simulink model "arlht_1920_1080"  (R2020a)
settings: Solver=FixedStepDiscrete  StartTime=0.0  StopTime=inf  RelTol=1e-3
InitFcn:
  | setup_parallel_hough_transform;
StopFcn:
  | %stop_parallel_hough_accumulator;
values from neighbouring files (symbols this model uses):
  bitsRho = ceil(log2(maxRho*2))    [setup_parallel_hough_transform.m]
  gamma = (179+1)/Ktheta    (= 45)    [setup_parallel_hough_transform.m]
  height = 1080    [setup_parallel_hough_transform.m]
  inarray = Y    [setup_parallel_hough_transform.m]
  Ktheta = 4    [setup_parallel_hough_transform.m]
  maxRho = ceil(sqrt((height/2)^2+(width/2)^2))    [setup_parallel_hough_transform.m]
  width = 1920    [setup_parallel_hough_transform.m]
undefined symbols (not defined in the file or in its folder): nTheta
libraries: simulink x27, hdlsllib x27, dspsrcs4 x1, dsphdlmathfun x1
(part 1 of 2)
settings Model: DataTypeOverride=Off  SimulationMode=rapid-accelerator  Creator=david  LastModifiedBy=david
settings OptimizationCC: BlockReduction=off  ConditionallyExecuteInputs=off  DefaultParameterBehavior=Inlined
settings DebuggingCC: AlgebraicLoopMsg=error  SingleTaskRateTransMsg=error
settings HardwareCC: ProdBitPerPointer=32  ProdBitPerSizeT=32  ProdBitPerPtrDiffT=32  ProdLargestAtomicFloat=None  ProdIntDivRoundTo=Undefined  ProdEndianess=Unspecified  ProdWordSize=32  ProdHWDeviceType=ASIC/FPGA->ASIC/FPGA  TargetBitPerPointer=64  TargetBitPerSizeT=64  TargetBitPerPtrDiffT=64  TargetLongLongMode=on  TargetIntDivRoundTo=Zero  TargetEndianess=LittleEndian  TargetWordSize=64  TargetHWDeviceType=Custom Processor->MATLAB Host Computer  ProdEqTarget=off

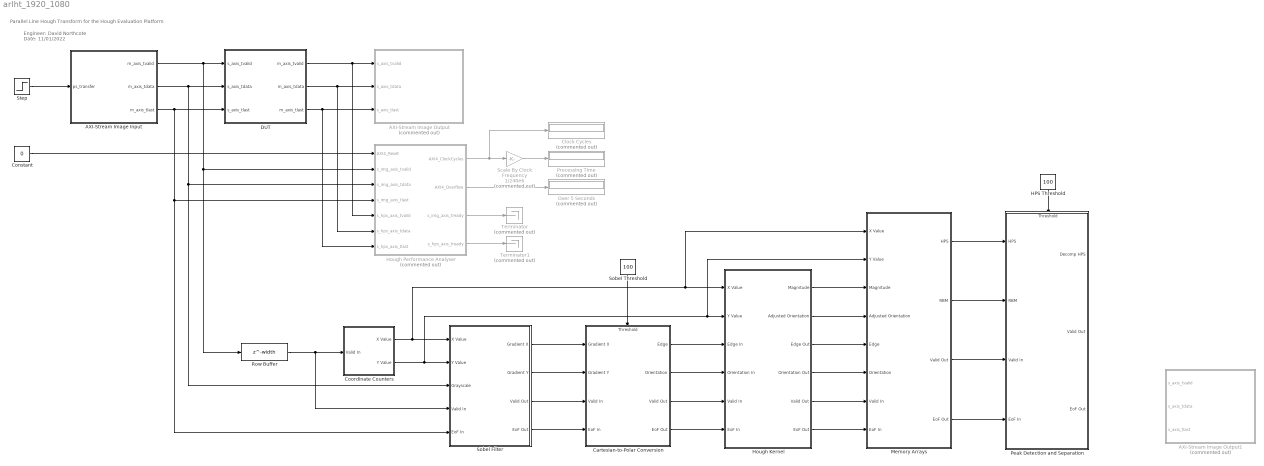
== system arlht_1920_1080 ==
  note: Engineer: David Northcote
      | Date: 11/01/2022
  note: Parallel Line Hough Transform for the Hough Evaluation Platform
  AXI-Stream Image Input : Subsystem  mask{image=inarray, clk=1/150e6}
      mask prompts: image "Input Image:"; clk "Clock Rate:"
      mask init:
      | [height, width] = size(image);
      mask DialogControl DescGroupVar Prompt: AXI-Stream Image Input
      mask DialogControl DescTextVar Prompt: This block simulates an AXI-Stream image input for interfacing to a hardware accelerator or IP Core.
      mask DialogControl ParameterGroupVar Prompt: Main
  AXI-Stream Image Output : Subsystem  Commented=on  mask{height=ceil(sqrt((height/2)^2+(width/2)^2))*2, width=numel([0:1:179]), clk=1/150e6, d=0}
      mask prompts: height "Image Height:"; width "Image Width:"; clk "Clock Rate:"; d "Frame Capture Number"
      mask DialogControl DescGroupVar Prompt: AXI-Stream Image Output
      mask DialogControl DescTextVar Prompt: Image output using the AXI-Stream interface. Simulates an AXI DMA write channel.
      mask DialogControl ParameterGroupVar Prompt: Main
  AXI-Stream Image Output1 : Subsystem  Commented=on  mask{height=height, width=width, clk=1/150e6, d=0}
      mask prompts: height "Image Height:"; width "Image Width:"; clk "Clock Rate:"; d "Frame Capture Number"
      mask DialogControl DescGroupVar Prompt: AXI-Stream Image Output
      mask DialogControl DescTextVar Prompt: Image output using the AXI-Stream interface. Simulates an AXI DMA write channel.
      mask DialogControl ParameterGroupVar Prompt: Main
  Cartesian-to-Polar Conversion : Subsystem
      settings: PortSchema="{\"entries\":[{\"content\":{\"sides\":[{\"content\":{\"connectorIds\":[\"In1\",\"In2\",\"In3\",\"In4\"]},\"type\":\"ConnectorPlacement.EquallySpacedRectSide\",\"uuid\":\"a3c8f507-c537-40f1-9a8a-bf401aec1e83\"},{\"content\":{\"connectorIds\":[\"Out1\",\"Out2\",\"Out3\",\"Out4\"],\"side\":\"RIGHT\"},\"type\":\"ConnectorPlacement.EquallySpacedRectSide\",\"uuid\":\"71853828-b65c-4dcd-97ef-062e77f4992b\"},{\"content\":{\"connectorIds\":[\"In5\"],\"side\":\"TOP\"},\"type\":\"ConnectorPlacement.EquallySpacedRectSide\",\"uuid\":\"70d50e18-3706-4f3a-b062-ad028f7ac4e8\"}]},\"type\":\"ConnectorPlacement.EquallySpacedConnector\",\"uuid\":\"ca8aacb5-c0af-4164-af92-5b8669b0f313\"}],\"packageUris\":[\"http://schema.mathworks.com/mf0/Connector/19700101\"],\"version\":\"1.0\"}"
  Clock Cycles : Display  Commented=on
  Constant : Constant  Value=0  OutDataTypeStr=boolean  SampleTime=1/150e6
  Coordinate Counters : Subsystem
  DUT : Subsystem  TreatAsAtomicUnit=on
  HPS Threshold : Constant  Value=100  OutDataTypeStr=uint8  SampleTime=-1
  Hough Kernel : Subsystem
  Hough Performance Analyser : Subsystem  Commented=on  TreatAsAtomicUnit=on
  Memory Arrays : Subsystem
  Over 5 Seconds : Display  Commented=on
  Peak Detection and Separation : Subsystem
      settings: PortSchema="{\"entries\":[{\"content\":{\"sides\":[{\"content\":{\"connectorIds\":[\"In1\",\"In2\",\"In3\",\"In4\"]},\"type\":\"ConnectorPlacement.EquallySpacedRectSide\",\"uuid\":\"a3c8f507-c537-40f1-9a8a-bf401aec1e83\"},{\"content\":{\"connectorIds\":[\"Out1\",\"Out2\",\"Out3\"],\"side\":\"RIGHT\"},\"type\":\"ConnectorPlacement.EquallySpacedRectSide\",\"uuid\":\"71853828-b65c-4dcd-97ef-062e77f4992b\"},{\"content\":{\"connectorIds\":[\"In5\"],\"side\":\"TOP\"},\"type\":\"ConnectorPlacement.EquallySpacedRectSide\",\"uuid\":\"70d50e18-3706-4f3a-b062-ad028f7ac4e8\"}]},\"type\":\"ConnectorPlacement.EquallySpacedConnector\",\"uuid\":\"ca8aacb5-c0af-4164-af92-5b8669b0f313\"}],\"packageUris\":[\"http://schema.mathworks.com/mf0/Connector/19700101\"],\"version\":\"1.0\"}"
  Processing Time : Display  Commented=on
  Row Buffer : Delay  DelayLength=width
  Scale By Clock Frequency : Gain  Commented=on  Gain=1/240e6  ParamDataTypeStr=double  OutDataTypeStr=double
  Sobel Filter : Subsystem
  Sobel Threshold : Constant  Value=100  OutDataTypeStr=uint8  SampleTime=-1
  Step : Step  Time=2/150e6  SampleTime=1/150e6
  Terminator : Terminator  Commented=on
  Terminator1 : Terminator  Commented=on
  wires:
  Hough Performance Analyser/1(AXI4_ClockCycles) -> Clock Cycles/1, Scale By Clock Frequency/1
  Scale By Clock Frequency/1 -> Processing Time/1
  DUT/3(m_axis_tlast) -> Hough Performance Analyser/7(s_hps_axis_tlast), AXI-Stream Image Output/3(s_axis_tlast)
  DUT/2(m_axis_tdata) -> Hough Performance Analyser/6(s_hps_axis_tdata), AXI-Stream Image Output/2(s_axis_tdata)
  DUT/1(m_axis_tvalid) -> Hough Performance Analyser/5(s_hps_axis_tvalid), AXI-Stream Image Output/1(s_axis_tvalid)
  AXI-Stream Image Input/3(m_axis_tlast) -> Sobel Filter/5(EoF In), Hough Performance Analyser/4(s_img_axis_tlast), DUT/3(s_axis_tlast)
  AXI-Stream Image Input/1(m_axis_tvalid) -> Row Buffer/1, Hough Performance Analyser/2(s_img_axis_tvalid), DUT/1(s_axis_tvalid)
  AXI-Stream Image Input/2(m_axis_tdata) -> Sobel Filter/3(Grayscale), Hough Performance Analyser/3(s_img_axis_tdata), DUT/2(s_axis_tdata)
  Hough Performance Analyser/2(AXI4_Overflow) -> Over 5 Seconds/1
  Constant/1 -> Hough Performance Analyser/1(AXI4_Reset)
  Step/1 -> AXI-Stream Image Input/1(ps_transfer)
  Hough Performance Analyser/4(s_hps_axis_tready) -> Terminator1/1
  Hough Performance Analyser/3(s_img_axis_tready) -> Terminator/1
  Coordinate Counters/2(Y Value) -> Memory Arrays/2(Y Value), Hough Kernel/2(Y Value), Sobel Filter/2(Y Value)
  Coordinate Counters/1(X Value) -> Hough Kernel/1(X Value), Memory Arrays/1(X Value), Sobel Filter/1(X Value)
  Row Buffer/1 -> Coordinate Counters/1(Valid In), Sobel Filter/4(Valid In)
  Sobel Filter/3(Valid Out) -> Cartesian-to-Polar Conversion/3(Valid In)
  Sobel Filter/4(EoF Out) -> Cartesian-to-Polar Conversion/4(EoF In)
  Sobel Filter/1(Gradient X) -> Cartesian-to-Polar Conversion/1(Gradient X)
  Sobel Filter/2(Gradient Y) -> Cartesian-to-Polar Conversion/2(Gradient Y)
  Cartesian-to-Polar Conversion/1(Edge) -> Hough Kernel/3(Edge In)
  Cartesian-to-Polar Conversion/2(Orientation) -> Hough Kernel/4(Orientation In)
  Cartesian-to-Polar Conversion/3(Valid Out) -> Hough Kernel/5(Valid In)
  Cartesian-to-Polar Conversion/4(EoF Out) -> Hough Kernel/6(EoF In)
  Hough Kernel/3(Edge Out) -> Memory Arrays/5(Edge)
  Hough Kernel/1(Magnitude) -> Memory Arrays/3(Magnitude)
  Hough Kernel/2(Adjusted Orientation) -> Memory Arrays/4(Adjusted Orientation)
  Hough Kernel/5(Valid Out) -> Memory Arrays/7(Valid In)
  Hough Kernel/6(EoF Out) -> Memory Arrays/8(EoF In)
  Sobel Threshold/1 -> Cartesian-to-Polar Conversion/5(Threshold)
  Memory Arrays/4(EoF Out) -> Peak Detection and Separation/4(EoF In)
  Memory Arrays/3(Valid Out) -> Peak Detection and Separation/3(Valid In)
  Memory Arrays/2(RBM) -> Peak Detection and Separation/2(RBM)
  Memory Arrays/1(HPS) -> Peak Detection and Separation/1(HPS)
  HPS Threshold/1 -> Peak Detection and Separation/5(Threshold)
  Hough Kernel/4(Orientation Out) -> Memory Arrays/6(Orientation)

== system arlht_1920_1080/AXI-Stream Image Input ==
  ps_transfer : Inport
  Compare To Constant : simulink/Logic and Bit Operations/Compare To Constant  relop===  const=height*width-1  OutDataTypeStr=boolean
  Constant : Constant  OutDataTypeStr=boolean  SampleTime=-1
  Data Type Conversion : DataTypeConversion  OutDataTypeStr=uint32
  HDL Counter : hdlsllib/Sources/HDL Counter  CountType=Free running  CountInit=0  CountStep=1  CountMax=width*height-1  CountFromType=Initial value  CountFrom=0  CountResetPort=on  CountLoadPort=off  CountEnbPort=on  CountDirPort=off  CountDataType=Unsigned  CountWordLen=32  CountFracLen=0  CountSampTime=1
  Multiport Switch : MultiPortSwitch  DataPortOrder=Zero-based contiguous  Inputs=2  zeroidx=on
  Rising Edge Detector : Subsystem
  Synchronous Image Source : Subsystem
  Unit Delay Resettable Synchronous : hdlsllib/Discrete/Unit Delay Resettable Synchronous  InitialCondition=0.0  SampleTime=-1
      settings: SourceProductBaseCode=SL
  m_axis_tvalid : Outport
  m_axis_tdata : Outport  Port=2
  m_axis_tlast : Outport  Port=3
  wires:
  Constant/1 -> Multiport Switch/3
  Rising Edge Detector/1(Output) -> Multiport Switch/1
  Unit Delay Resettable Synchronous/1 -> Multiport Switch/2
  ps_transfer/1 -> Rising Edge Detector/1(Input)
  Data Type Conversion/1 -> m_axis_tdata/1
  Compare To Constant/1 -> m_axis_tlast/1, HDL Counter/1, Unit Delay Resettable Synchronous/2
  Multiport Switch/1 -> m_axis_tvalid/1, Synchronous Image Source/Enable, HDL Counter/2, Unit Delay Resettable Synchronous/1
  Synchronous Image Source/1(Pixel) -> Data Type Conversion/1
  HDL Counter/1 -> Compare To Constant/1

== system arlht_1920_1080/AXI-Stream Image Output ==
  s_axis_tvalid : Inport
  s_axis_tdata : Inport  Port=2
  s_axis_tlast : Inport  Port=3
  Delay : Delay  DelayLength=4
  Delay1 : Delay  DelayLength=d  ShowEnablePort=on
      settings: InputPortMap=u0,e6
  Pixel to Workspace : Subsystem
  Stop Simulation2 : Stop
  wires:
  Delay/1 -> Stop Simulation2/1
  Delay1/1 -> Delay/1
  s_axis_tlast/1 -> Delay1/1, Delay1/2
  s_axis_tdata/1 -> Pixel to Workspace/1(Pixel In)
  s_axis_tvalid/1 -> Pixel to Workspace/Enable

== system arlht_1920_1080/AXI-Stream Image Output1 ==
  s_axis_tvalid : Inport
  s_axis_tdata : Inport  Port=2
  s_axis_tlast : Inport  Port=3
  Delay : Delay  DelayLength=4
  Delay1 : Delay  DelayLength=d  ShowEnablePort=on
      settings: InputPortMap=u0,e6
  Pixel to Workspace : Subsystem
  Stop Simulation2 : Stop
  wires:
  s_axis_tvalid/1 -> Pixel to Workspace/Enable
  s_axis_tdata/1 -> Pixel to Workspace/1(Pixel In)
  s_axis_tlast/1 -> Delay1/2, Delay1/1
  Delay1/1 -> Delay/1
  Delay/1 -> Stop Simulation2/1

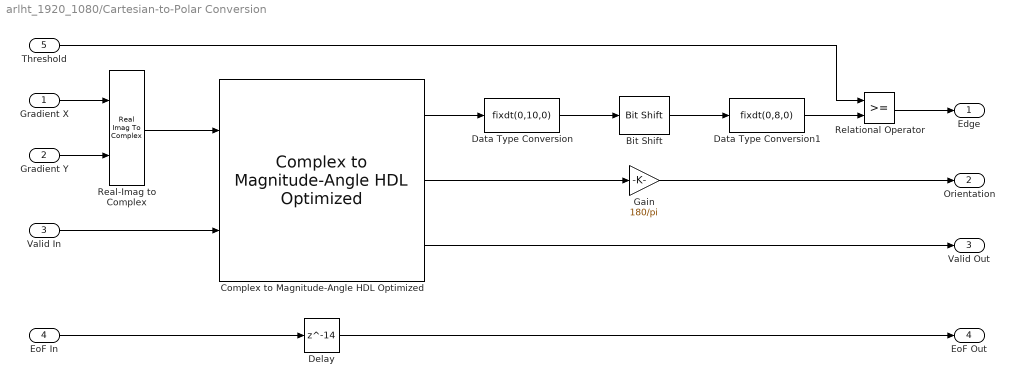
== system arlht_1920_1080/Cartesian-to-Polar Conversion ==
  Gradient X : Inport
  Gradient Y : Inport  Port=2
  Valid In : Inport  Port=3
  EoF In : Inport  Port=4
  Threshold : Inport  Port=5
  Bit Shift : hdlsllib/Logic and Bit Operations/Bit Shift  mode=Shift Right Logical  N=2
  Complex to Magnitude-Angle HDL Optimized : dsphdlmathfun/Complex to Magnitude-Angle HDL Optimized  NumIterationsSource=Property  NumIterations=9  OutputFormat=Magnitude and angle  AngleFormat=Radians  ScaleOutput=on  SimulateUsing=Code generation
      settings: SourceProductBaseCode=DS
  Data Type Conversion : DataTypeConversion  OutDataTypeStr=fixdt(0,10,0)  SaturateOnIntegerOverflow=on
  Data Type Conversion1 : DataTypeConversion  OutDataTypeStr=fixdt(0,8,0)  SaturateOnIntegerOverflow=on
  Delay : Delay  DelayLength=14
  Gain : Gain  Gain=180/pi  ParamDataTypeStr=fixdt(0,16,16-6)  OutDataTypeStr=uint8  RndMeth=Round
  Real-Imag to Complex : RealImagToComplex
  Relational Operator : RelationalOperator  OutDataTypeStr=boolean  RndMeth=Simplest
  Edge : Outport
  Orientation : Outport  Port=2
  Valid Out : Outport  Port=3
  EoF Out : Outport  Port=4
  wires:
  Real-Imag to Complex/1 -> Complex to Magnitude-Angle HDL Optimized/1
  Valid In/1 -> Complex to Magnitude-Angle HDL Optimized/2
  EoF In/1 -> Delay/1
  Complex to Magnitude-Angle HDL Optimized/3 -> Valid Out/1
  Delay/1 -> EoF Out/1
  Gradient X/1 -> Real-Imag to Complex/1
  Gradient Y/1 -> Real-Imag to Complex/2
  Complex to Magnitude-Angle HDL Optimized/1 -> Data Type Conversion/1
  Data Type Conversion/1 -> Bit Shift/1
  Bit Shift/1 -> Data Type Conversion1/1
  Complex to Magnitude-Angle HDL Optimized/2 -> Gain/1
  Gain/1 -> Orientation/1
  Data Type Conversion1/1 -> Relational Operator/2
  Relational Operator/1 -> Edge/1
  Threshold/1 -> Relational Operator/1

== system arlht_1920_1080/Coordinate Counters ==
  Valid In : Inport
  AND : Logic  IconShape=distinctive  AllPortsSameDT=off  OutDataTypeStr=boolean
  Compare To Constant : simulink/Logic and Bit Operations/Compare To Constant  relop===  const=width/2-1  OutDataTypeStr=boolean
  X Counter : hdlsllib/Sources/HDL Counter  CountType=Count limited  CountInit=-width/2  CountStep=1  CountMax=width/2-1  CountFromType=Initial value  CountFrom=-width/2  CountResetPort=off  CountLoadPort=off  CountEnbPort=on  CountDirPort=off  CountDataType=Signed  CountWordLen=ceil(log2(width/2)) + 1  CountFracLen=0  CountSampTime=1
  Y Counter : hdlsllib/Sources/HDL Counter  CountType=Count limited  CountInit=-height/2  CountStep=1  CountMax=height/2-1  CountFromType=Initial value  CountFrom=-height/2  CountResetPort=off  CountLoadPort=off  CountEnbPort=on  CountDirPort=off  CountDataType=Signed  CountWordLen=ceil(log2(height/2)) + 1  CountFracLen=0  CountSampTime=1
  X Value : Outport  VectorParamsAs1DForOutWhenUnconnected=off
  Y Value : Outport  Port=2  VectorParamsAs1DForOutWhenUnconnected=off
  wires:
  Valid In/1 -> AND/2, X Counter/1
  X Counter/1 -> X Value/1, Compare To Constant/1
  Y Counter/1 -> Y Value/1
  AND/1 -> Y Counter/1
  Compare To Constant/1 -> AND/1

== system arlht_1920_1080/DUT ==
  s_axis_tvalid : Inport
  s_axis_tdata : Inport  Port=2
  s_axis_tlast : Inport  Port=3
  LHT : Subsystem
  m_axis_tvalid : Outport  VectorParamsAs1DForOutWhenUnconnected=off
  m_axis_tdata : Outport  Port=2  VectorParamsAs1DForOutWhenUnconnected=off
  m_axis_tlast : Outport  Port=3  VectorParamsAs1DForOutWhenUnconnected=off
  wires:
  s_axis_tdata/1 -> LHT/1(s_tdata)
  s_axis_tvalid/1 -> LHT/2(s_tvalid)
  s_axis_tlast/1 -> LHT/3(s_tlast)
  LHT/3(m_axis_tlast) -> m_axis_tlast/1
  LHT/1(m_axis_tdata) -> m_axis_tdata/1
  LHT/2(m_axis_tvalid) -> m_axis_tvalid/1

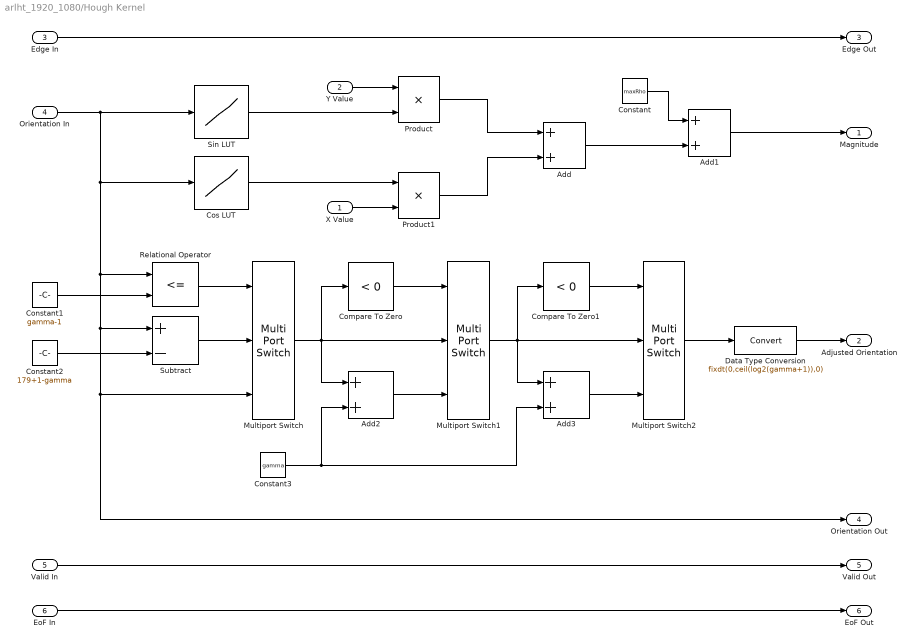
== system arlht_1920_1080/Hough Kernel ==
  X Value : Inport
  Y Value : Inport  Port=2
  Edge In : Inport  Port=3
  Orientation In : Inport  Port=4
  Valid In : Inport  Port=5
  EoF In : Inport  Port=6
  Add : Sum
  Add1 : Sum  OutDataTypeStr=fixdt(0,bitsRho,0)
  Add2 : Sum  OutDataTypeStr=Inherit: Same as first input
  Add3 : Sum  OutDataTypeStr=Inherit: Same as first input
  Compare To Zero : simulink/Logic and Bit Operations/Compare To Zero  relop=<  OutDataTypeStr=boolean
  Compare To Zero1 : simulink/Logic and Bit Operations/Compare To Zero  relop=<  OutDataTypeStr=boolean
  Constant : Constant  Value=maxRho  OutDataTypeStr=fixdt(0,ceil(log2(maxRho+1)),0)  SampleTime=-1
  Constant1 : Constant  Value=gamma-1  OutDataTypeStr=fixdt(0,ceil(log2(gamma)),0)  SampleTime=-1
  Constant2 : Constant  Value=179+1-gamma  OutDataTypeStr=fixdt(0,ceil(log2(179+1-gamma)),0)  SampleTime=-1
  Constant3 : Constant  Value=gamma  OutDataTypeStr=fixdt(0,ceil(log2(gamma+1)),0)  SampleTime=-1
  Cos LUT : Lookup_n-D  NumberOfTableDimensions=1  BreakpointsForDimension1=[0:1:179]  IndexSearchMethod=Evenly spaced points  Table=cos(deg2rad(0:1:179))  InterpMethod=Flat  DiagnosticForOutOfRangeInput=Error  InternalRulePriority=Speed  OutDataTypeStr=fixdt(1,16,14)  RndMeth=Simplest  InputSameDT=on
  Data Type Conversion : DataTypeConversion  OutDataTypeStr=fixdt(0,ceil(log2(gamma+1)),0)
  Multiport Switch : MultiPortSwitch  DataPortOrder=Zero-based contiguous  Inputs=2  zeroidx=on
  Multiport Switch1 : MultiPortSwitch  DataPortOrder=Zero-based contiguous  Inputs=2  zeroidx=on
  Multiport Switch2 : MultiPortSwitch  DataPortOrder=Zero-based contiguous  Inputs=2  zeroidx=on
  Product : Product  OutDataTypeStr=fixdt(1,ceil(log2(height)),0)  RndMeth=Round
  Product1 : Product  OutDataTypeStr=fixdt(1,ceil(log2(width)),0)  RndMeth=Round
  Relational Operator : RelationalOperator  Operator=<=  OutDataTypeStr=boolean  RndMeth=Simplest
  Sin LUT : Lookup_n-D  NumberOfTableDimensions=1  BreakpointsForDimension1=[0:1:179]  IndexSearchMethod=Evenly spaced points  Table=sin(deg2rad(0:1:179))  InterpMethod=Flat  DiagnosticForOutOfRangeInput=Error  InternalRulePriority=Speed  OutDataTypeStr=fixdt(1,16,14)  RndMeth=Simplest  InputSameDT=on
  Subtract : Sum  Inputs=+-
  Magnitude : Outport
  Adjusted Orientation : Outport  Port=2
  Edge Out : Outport  Port=3
  Orientation Out : Outport  Port=4
  Valid Out : Outport  Port=5
  EoF Out : Outport  Port=6
  wires:
  Valid In/1 -> Valid Out/1
  EoF In/1 -> EoF Out/1
  Edge In/1 -> Edge Out/1
  Sin LUT/1 -> Product/2
  Cos LUT/1 -> Product1/1
  Product/1 -> Add/1
  Product1/1 -> Add/2
  Y Value/1 -> Product/1
  X Value/1 -> Product1/2
  Orientation In/1 -> Sin LUT/1, Orientation Out/1, Multiport Switch/3, Subtract/1, Relational Operator/1, Cos LUT/1
  Add1/1 -> Magnitude/1
  Add/1 -> Add1/2
  Constant/1 -> Add1/1
  Relational Operator/1 -> Multiport Switch/1
  Constant1/1 -> Relational Operator/2
  Constant2/1 -> Subtract/2
  Constant3/1 -> Add3/2, Add2/2
  Multiport Switch/1 -> Add2/1, Compare To Zero/1, Multiport Switch1/2
  Add2/1 -> Multiport Switch1/3
  Compare To Zero/1 -> Multiport Switch1/1
  Subtract/1 -> Multiport Switch/2
  Compare To Zero1/1 -> Multiport Switch2/1
  Add3/1 -> Multiport Switch2/3
  Multiport Switch1/1 -> Add3/1, Compare To Zero1/1, Multiport Switch2/2
  Multiport Switch2/1 -> Data Type Conversion/1
  Data Type Conversion/1 -> Adjusted Orientation/1

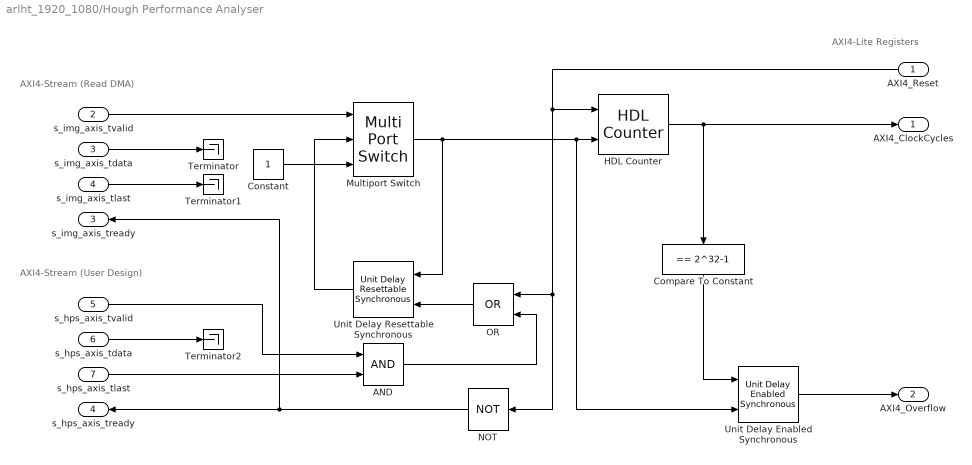
== system arlht_1920_1080/Hough Performance Analyser ==
  note: AXI4-Stream (Read DMA)
  note: AXI4-Stream (User Design)
  note: AXI4-Lite Registers
  AXI4_Reset : Inport
  s_img_axis_tvalid : Inport  Port=2
  s_img_axis_tdata : Inport  Port=3
  s_img_axis_tlast : Inport  Port=4
  s_hps_axis_tvalid : Inport  Port=5
  s_hps_axis_tdata : Inport  Port=6
  s_hps_axis_tlast : Inport  Port=7
  AND : Logic  IconShape=distinctive  AllPortsSameDT=off  OutDataTypeStr=boolean
  Compare To Constant : simulink/Logic and Bit Operations/Compare To Constant  relop===  const=2^32-1  OutDataTypeStr=boolean
  Constant : Constant  OutDataTypeStr=boolean  SampleTime=-1
  HDL Counter : hdlsllib/Sources/HDL Counter  CountType=Count limited  CountInit=0  CountStep=1  CountMax=2^32-1  CountFromType=Initial value  CountFrom=0  CountResetPort=on  CountLoadPort=off  CountEnbPort=on  CountDirPort=off  CountDataType=Unsigned  CountWordLen=32  CountFracLen=0  CountSampTime=1
  Multiport Switch : MultiPortSwitch  DataPortOrder=Zero-based contiguous  Inputs=2  zeroidx=on
  NOT : Logic  Operator=NOT  IconShape=distinctive  AllPortsSameDT=off  OutDataTypeStr=boolean
  OR : Logic  Operator=OR  IconShape=distinctive  AllPortsSameDT=off  OutDataTypeStr=boolean
  Terminator : Terminator
  Terminator1 : Terminator
  Terminator2 : Terminator
  Unit Delay Enabled Synchronous : hdlsllib/Discrete/Unit Delay Enabled Synchronous  InitialCondition=0.0  SampleTime=-1
      settings: SourceProductBaseCode=SL
  Unit Delay Resettable Synchronous : hdlsllib/Discrete/Unit Delay Resettable Synchronous  InitialCondition=0.0  SampleTime=-1
      settings: SourceProductBaseCode=SL
  AXI4_ClockCycles : Outport
  AXI4_Overflow : Outport  Port=2
  s_img_axis_tready : Outport  Port=3
  s_hps_axis_tready : Outport  Port=4
  wires:
  NOT/1 -> s_hps_axis_tready/1, s_img_axis_tready/1
  s_hps_axis_tvalid/1 -> AND/1
  s_hps_axis_tlast/1 -> AND/2
  AND/1 -> OR/2
  s_img_axis_tvalid/1 -> Multiport Switch/1
  OR/1 -> Unit Delay Resettable Synchronous/2
  s_img_axis_tlast/1 -> Terminator1/1
  AXI4_Reset/1 -> HDL Counter/1, OR/1, NOT/1
  s_img_axis_tdata/1 -> Terminator/1
  s_hps_axis_tdata/1 -> Terminator2/1
  HDL Counter/1 -> AXI4_ClockCycles/1, Compare To Constant/1
  Unit Delay Enabled Synchronous/1 -> AXI4_Overflow/1
  Compare To Constant/1 -> Unit Delay Enabled Synchronous/1
  Multiport Switch/1 -> HDL Counter/2, Unit Delay Enabled Synchronous/2, Unit Delay Resettable Synchronous/1
  Unit Delay Resettable Synchronous/1 -> Multiport Switch/2
  Constant/1 -> Multiport Switch/3

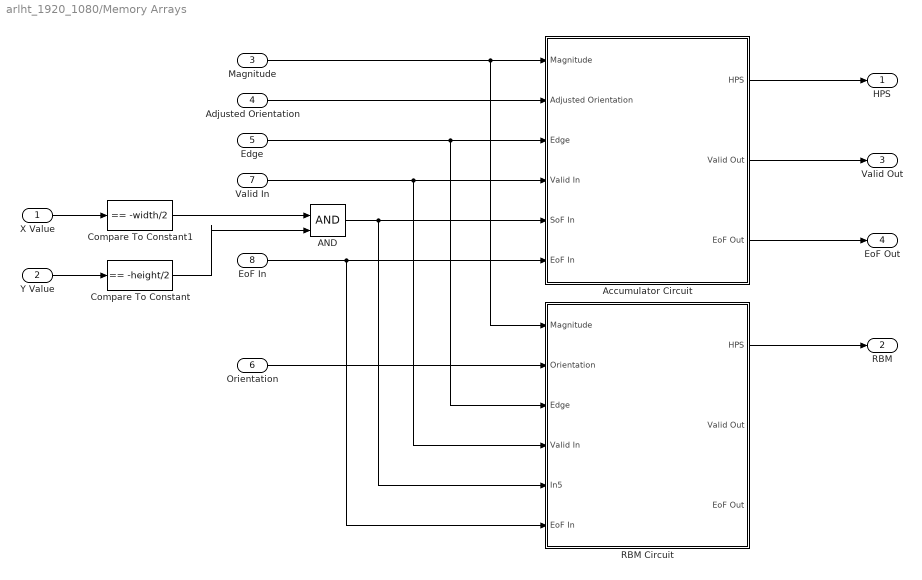
== system arlht_1920_1080/Memory Arrays ==
  X Value : Inport
  Y Value : Inport  Port=2
  Magnitude : Inport  Port=3
  Adjusted Orientation : Inport  Port=4
  Edge : Inport  Port=5
  Orientation : Inport  Port=6
  Valid In : Inport  Port=7
  EoF In : Inport  Port=8
  AND : Logic  IconShape=distinctive  AllPortsSameDT=off  OutDataTypeStr=boolean
  Accumulator Circuit : Subsystem
  Compare To Constant : simulink/Logic and Bit Operations/Compare To Constant  relop===  const=-height/2  OutDataTypeStr=boolean
  Compare To Constant1 : simulink/Logic and Bit Operations/Compare To Constant  relop===  const=-width/2  OutDataTypeStr=boolean
  RBM Circuit : Subsystem
  HPS : Outport
  RBM : Outport  Port=2
  Valid Out : Outport  Port=3
  EoF Out : Outport  Port=4
  wires:
  Magnitude/1 -> RBM Circuit/1(Magnitude), Accumulator Circuit/1(Magnitude)
  Adjusted Orientation/1 -> Accumulator Circuit/2(Adjusted Orientation)
  Edge/1 -> RBM Circuit/3(Edge), Accumulator Circuit/3(Edge)
  Valid In/1 -> RBM Circuit/4(Valid In), Accumulator Circuit/4(Valid In)
  EoF In/1 -> RBM Circuit/6(EoF In), Accumulator Circuit/6(EoF In)
  Accumulator Circuit/1(HPS) -> HPS/1
  RBM Circuit/1(HPS) -> RBM/1
  Accumulator Circuit/2(Valid Out) -> Valid Out/1
  Accumulator Circuit/3(EoF Out) -> EoF Out/1
  Orientation/1 -> RBM Circuit/2(Orientation)
  Compare To Constant/1 -> AND/2
  Compare To Constant1/1 -> AND/1
  X Value/1 -> Compare To Constant1/1
  Y Value/1 -> Compare To Constant/1
  AND/1 -> RBM Circuit/5(In5), Accumulator Circuit/5(SoF In)

== system arlht_1920_1080/Peak Detection and Separation ==
  HPS : Inport
  RBM : Inport  Port=2
  Valid In : Inport  Port=3
  EoF In : Inport  Port=4
  Threshold : Inport  Port=5
  Decomp HPS : Outport
  Valid Out : Outport  Port=2
  EoF Out : Outport  Port=3
  wires:
  ? -> Decomp HPS/1

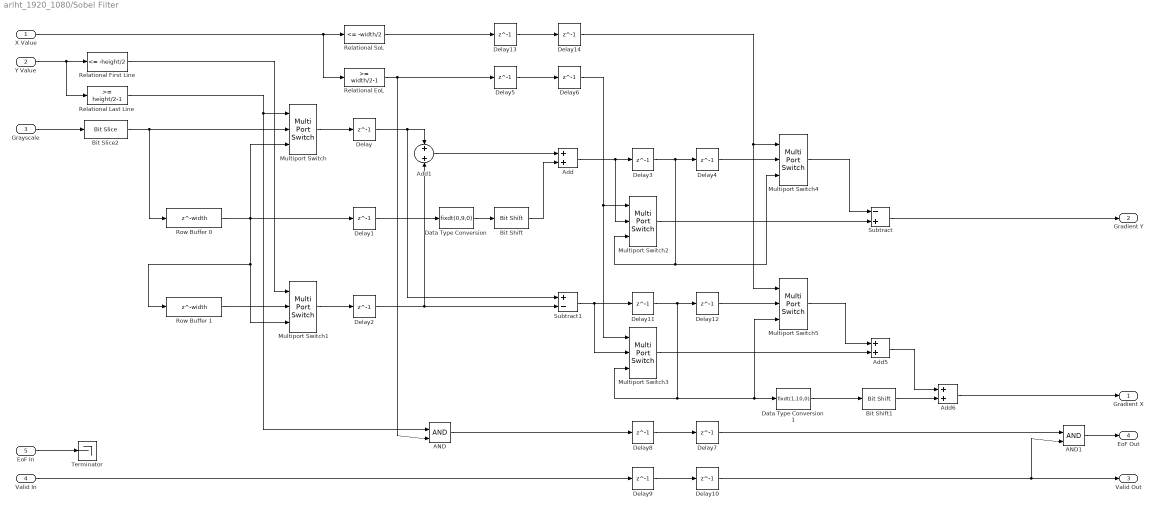
== system arlht_1920_1080/Sobel Filter ==
  X Value : Inport
  Y Value : Inport  Port=2
  Grayscale : Inport  Port=3
  Valid In : Inport  Port=4
  EoF In : Inport  Port=5
  AND : Logic  IconShape=distinctive  AllPortsSameDT=off  OutDataTypeStr=boolean
  AND1 : Logic  IconShape=distinctive  AllPortsSameDT=off  OutDataTypeStr=boolean
  Add{,1,5..6} (4 alike) : Sum
  Bit Shift : hdlsllib/Logic and Bit Operations/Bit Shift  mode=Shift Left Logical  N=1
  Bit Shift1 : hdlsllib/Logic and Bit Operations/Bit Shift  mode=Shift Left Logical  N=1
  Bit Slice2 : hdlsllib/Logic and Bit Operations/Bit Slice  lidx=7  ridx=0
      settings: SourceProductBaseCode=SL
  Data Type Conversion : DataTypeConversion  OutDataTypeStr=fixdt(0,9,0)
  Data Type Conversion1 : DataTypeConversion  OutDataTypeStr=fixdt(1,10,0)
  Delay{,1..14} (15 alike) : Delay  DelayLength=1
  Multiport Switch{,1..5} (6 alike) : MultiPortSwitch  DataPortOrder=Zero-based contiguous  Inputs=2  zeroidx=on
  Relational EoL : simulink/Logic and Bit Operations/Compare To Constant  relop=>=  const=width/2-1  OutDataTypeStr=boolean
  Relational First Line : simulink/Logic and Bit Operations/Compare To Constant  relop=<=  const=-height/2  OutDataTypeStr=boolean
  Relational Last Line : simulink/Logic and Bit Operations/Compare To Constant  relop=>=  const=height/2-1  OutDataTypeStr=boolean
  Relational SoL : simulink/Logic and Bit Operations/Compare To Constant  relop=<=  const=-width/2  OutDataTypeStr=boolean
  Row Buffer 0 : Delay  DelayLength=width
  Row Buffer 1 : Delay  DelayLength=width
  Subtract : Sum  Inputs=-+
  Subtract1 : Sum  Inputs=+-
  Terminator : Terminator
  Gradient X : Outport
  Gradient Y : Outport  Port=2
  Valid Out : Outport  Port=3
  EoF Out : Outport  Port=4
  wires:
  Grayscale/1 -> Bit Slice2/1
  Bit Slice2/1 -> Multiport Switch/2, Row Buffer 0/1
  EoF In/1 -> Terminator/1
  Add6/1 -> Gradient X/1
  Delay8/1 -> Delay7/1
  AND/1 -> Delay8/1
  Valid In/1 -> Delay9/1
  Delay9/1 -> Delay10/1
  Delay10/1 -> AND1/2, Valid Out/1
  Delay3/1 -> Multiport Switch2/3, Multiport Switch4/3, Delay4/1
  Data Type Conversion/1 -> Bit Shift/1
  Delay/1 -> Add1/1, Subtract1/1
  Add1/1 -> Add/1
  Delay1/1 -> Data Type Conversion/1
  Subtract/1 -> Gradient Y/1
  Delay2/1 -> Subtract1/2, Add1/2
  Delay11/1 -> Delay12/1, Multiport Switch3/3, Data Type Conversion1/1, Multiport Switch5/3
  Add5/1 -> Add6/1
  Bit Shift1/1 -> Add6/2
  Y Value/1 -> Relational Last Line/1, Relational First Line/1
  X Value/1 -> Relational EoL/1, Relational SoL/1
  Multiport Switch/1 -> Delay/1
  Relational Last Line/1 -> AND/1, Multiport Switch/1
  Multiport Switch1/1 -> Delay2/1
  Relational First Line/1 -> Multiport Switch1/1
  Row Buffer 0/1 -> Row Buffer 1/1, Multiport Switch1/3, Delay1/1, Multiport Switch/3
  Row Buffer 1/1 -> Multiport Switch1/2
  Multiport Switch2/1 -> Subtract/2
  Add/1 -> Delay3/1, Multiport Switch2/2
  Subtract1/1 -> Delay11/1, Multiport Switch3/2
  Multiport Switch3/1 -> Add5/2
  Relational EoL/1 -> AND/2, Delay5/1
  Delay5/1 -> Delay6/1
  Delay6/1 -> Multiport Switch2/1, Multiport Switch3/1
  Delay4/1 -> Multiport Switch4/2
  Multiport Switch4/1 -> Subtract/1
  Delay12/1 -> Multiport Switch5/2
  Multiport Switch5/1 -> Add5/1
  Relational SoL/1 -> Delay13/1
  Delay13/1 -> Delay14/1
  Delay14/1 -> Multiport Switch5/1, Multiport Switch4/1
  Delay7/1 -> AND1/1
  AND1/1 -> EoF Out/1
  Bit Shift/1 -> Add/2
  Data Type Conversion1/1 -> Bit Shift1/1

== system arlht_1920_1080/AXI-Stream Image Input/Rising Edge Detector ==
  Input : Inport
  AND : Logic  IconShape=distinctive  AllPortsSameDT=off  OutDataTypeStr=boolean
  Delay : Delay  DelayLength=1
  NOT : Logic  Operator=NOT  IconShape=distinctive  AllPortsSameDT=off  OutDataTypeStr=boolean
  Output : Outport  VectorParamsAs1DForOutWhenUnconnected=off
  wires:
  AND/1 -> Output/1
  Delay/1 -> AND/1
  Input/1 -> NOT/1, AND/2
  NOT/1 -> Delay/1

== system arlht_1920_1080/AXI-Stream Image Input/Synchronous Image Source ==
  Enable : EnablePort
  Signal From Workspace : dspsrcs4/Signal From Workspace  X=reshape(image', [height*width, 1])  Ts=clk  nsamps=1  OutputAfterFinalValue=Cyclic repetition  ignoreOrWarnInputAndFrameLengths=off  OutputFrames=off
  Pixel : Outport
  wires:
  Signal From Workspace/1 -> Pixel/1

== system arlht_1920_1080/AXI-Stream Image Output/Pixel to Workspace ==
  Pixel In : Inport
  Enable : EnablePort
  To Workspace : ToWorkspace  VariableName=simout  SampleTime=-1
      settings: MaxDataPoints=height*width  Save2DSignal=2-D array (concatenate along first dimension)
  wires:
  Pixel In/1 -> To Workspace/1

== system arlht_1920_1080/AXI-Stream Image Output1/Pixel to Workspace ==
  Pixel In : Inport
  Enable : EnablePort
  To Workspace : ToWorkspace  VariableName=simout  SampleTime=-1
      settings: MaxDataPoints=height*width  Save2DSignal=2-D array (concatenate along first dimension)
  wires:
  Pixel In/1 -> To Workspace/1

== system arlht_1920_1080/DUT/LHT ==
  s_tdata : Inport
  s_tvalid : Inport  Port=2
  s_tlast : Inport  Port=3
  Data Type Conversion : DataTypeConversion  Commented=on  OutDataTypeStr=uint32
  Parallel LHT Accumulator : Subsystem  Commented=on  mask{height=height, width=width, theta=[0:1:179]}
      mask prompts: height "Image Height:"; width "Image Width:"; theta "Orientations:"
      mask init:
      | maxRho = ceil(sqrt((height/2)^2+(width/2)^2));
      | nRho = maxRho*2;
      | [~, nTheta] = size(theta);
      mask DialogControl ParameterGroupVar Prompt: Main
  Parallel LHT Kernel : Subsystem  Commented=on
  m_axis_tdata : Outport  VectorParamsAs1DForOutWhenUnconnected=off
  m_axis_tvalid : Outport  Port=2  VectorParamsAs1DForOutWhenUnconnected=off
  m_axis_tlast : Outport  Port=3  VectorParamsAs1DForOutWhenUnconnected=off
  wires:
  s_tdata/1 -> Parallel LHT Kernel/1(s_tdata)
  s_tvalid/1 -> Parallel LHT Kernel/2(s_tvalid)
  s_tlast/1 -> Parallel LHT Kernel/3(s_tlast)
  Parallel LHT Kernel/1(m_axis_tvalid) -> Parallel LHT Accumulator/1(s_axis_tvalid)
  Parallel LHT Kernel/2(m_axis_tdata) -> Parallel LHT Accumulator/2(s_axis_tdata)
  Parallel LHT Kernel/4(m_axis_tlast) -> Parallel LHT Accumulator/4(s_axis_tlast)
  Parallel LHT Kernel/3(m_axis_tuser) -> Parallel LHT Accumulator/3(s_axis_tuser)
  Parallel LHT Kernel/5(hough_param) -> Parallel LHT Accumulator/5(hough_param)
  Parallel LHT Accumulator/2(m_axis_tdata) -> Data Type Conversion/1
  Parallel LHT Accumulator/1(m_axis_tvalid) -> m_axis_tvalid/1
  Parallel LHT Accumulator/3(m_axis_tlast) -> m_axis_tlast/1
  Data Type Conversion/1 -> m_axis_tdata/1

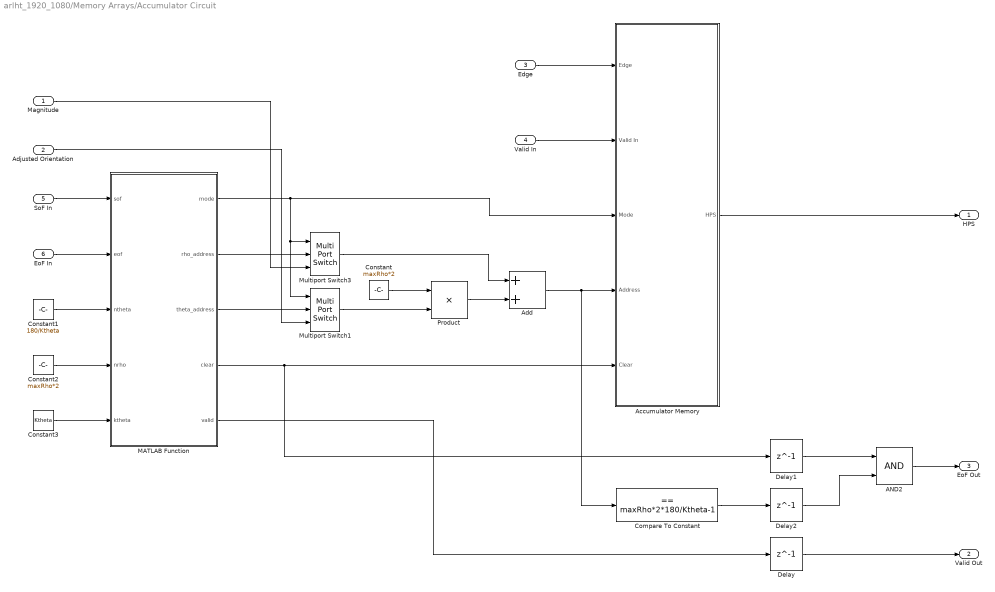
== system arlht_1920_1080/Memory Arrays/Accumulator Circuit ==
  Magnitude : Inport
  Adjusted Orientation : Inport  Port=2
  Edge : Inport  Port=3
  Valid In : Inport  Port=4
  SoF In : Inport  Port=5
  EoF In : Inport  Port=6
  AND2 : Logic  IconShape=distinctive  AllPortsSameDT=off  OutDataTypeStr=boolean
  Accumulator Memory : Subsystem
  Add : Sum  OutDataTypeStr=fixdt(0,ceil(log2(maxRho*2*45)),0)
  Compare To Constant : simulink/Logic and Bit Operations/Compare To Constant  relop===  const=maxRho*2*180/Ktheta-1  OutDataTypeStr=boolean
  Constant : Constant  Value=maxRho*2  OutDataTypeStr=fixdt(0,ceil(log2(maxRho*2+1)),0)  SampleTime=-1
  Constant1 : Constant  Value=180/Ktheta  OutDataTypeStr=uint8  SampleTime=-1
  Constant2 : Constant  Value=maxRho*2  OutDataTypeStr=uint16  SampleTime=-1
  Constant3 : Constant  Value=Ktheta  OutDataTypeStr=uint8  SampleTime=-1
  Delay : Delay  DelayLength=1  InitialCondition=0  UseCircularBuffer=on
  Delay1 : Delay  DelayLength=1  InitialCondition=0  UseCircularBuffer=on
  Delay2 : Delay  DelayLength=1  InitialCondition=0  UseCircularBuffer=on
  MATLAB Function : MATLAB Function  TreatAsAtomicUnit=on
  Multiport Switch1 : MultiPortSwitch  DataPortOrder=Zero-based contiguous  Inputs=2  zeroidx=on
  Multiport Switch3 : MultiPortSwitch  DataPortOrder=Zero-based contiguous  Inputs=2  zeroidx=on
  Product : Product  OutDataTypeStr=fixdt(0,ceil(log2(maxRho*2*44)),0)
  HPS : Outport
  Valid Out : Outport  Port=2
  EoF Out : Outport  Port=3
  wires:
  EoF In/1 -> MATLAB Function/2(eof)
  SoF In/1 -> MATLAB Function/1(sof)
  MATLAB Function/4(clear) -> Delay1/1, Accumulator Memory/5(Clear)
  MATLAB Function/5(valid) -> Delay/1
  Delay/1 -> Valid Out/1
  AND2/1 -> EoF Out/1
  Delay1/1 -> AND2/1
  Delay2/1 -> AND2/2
  Constant1/1 -> MATLAB Function/3(ntheta)
  Constant2/1 -> MATLAB Function/4(nrho)
  Constant3/1 -> MATLAB Function/5(ktheta)
  Compare To Constant/1 -> Delay2/1
  Magnitude/1 -> Multiport Switch3/3
  Adjusted Orientation/1 -> Multiport Switch1/3
  Edge/1 -> Accumulator Memory/1(Edge)
  Valid In/1 -> Accumulator Memory/2(Valid In)
  Accumulator Memory/1(HPS) -> HPS/1
  Add/1 -> Compare To Constant/1, Accumulator Memory/4(Address)
  Multiport Switch1/1 -> Product/2
  Multiport Switch3/1 -> Add/1
  Product/1 -> Add/2
  Constant/1 -> Product/1
  MATLAB Function/1(mode) -> Multiport Switch1/1, Multiport Switch3/1, Accumulator Memory/3(Mode)
  MATLAB Function/2(rho_address) -> Multiport Switch3/2
  MATLAB Function/3(theta_address) -> Multiport Switch1/2

== system arlht_1920_1080/Memory Arrays/RBM Circuit ==
  Magnitude : Inport
  Orientation : Inport  Port=2
  Edge : Inport  Port=3
  Valid In : Inport  Port=4
  In5 : Inport  Port=5
  EoF In : Inport  Port=6
  RBM Controller : Subsystem
  RBM Memory : Subsystem
  HPS : Outport
  Valid Out : Outport  Port=2
  EoF Out : Outport  Port=3
  wires:
  RBM Memory/1(hps) -> HPS/1
  RBM Controller/3(Out2) -> RBM Memory/3(enable)
  RBM Controller/2(y) -> RBM Memory/2(address)
  RBM Controller/1(Out1) -> RBM Memory/1(mode)
  RBM Controller/5(EoF Out) -> EoF Out/1
  RBM Controller/4(Valid Out) -> Valid Out/1
  EoF In/1 -> RBM Controller/5(EoF In)
  Valid In/1 -> RBM Controller/4(Valid In)
  Edge/1 -> RBM Controller/3(Edge)
  Orientation/1 -> RBM Controller/2(Adjusted Orientation)
  Magnitude/1 -> RBM Controller/1(Magnitude)

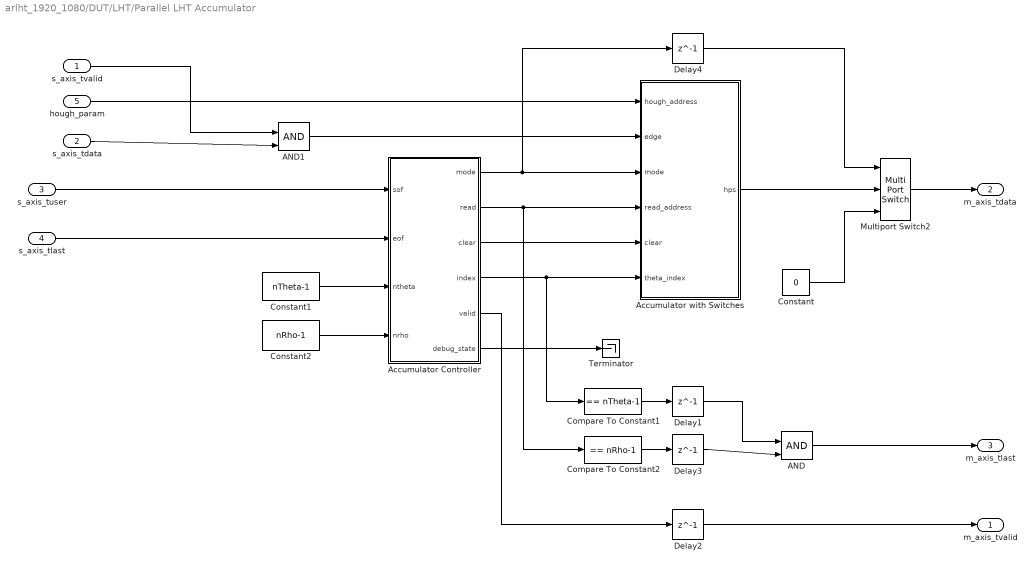
== system arlht_1920_1080/DUT/LHT/Parallel LHT Accumulator ==
  s_axis_tvalid : Inport
  s_axis_tdata : Inport  Port=2
  s_axis_tuser : Inport  Port=3
  s_axis_tlast : Inport  Port=4
  hough_param : Inport  Port=5
  AND : Logic  IconShape=distinctive  AllPortsSameDT=off  OutDataTypeStr=boolean
  AND1 : Logic  IconShape=distinctive  AllPortsSameDT=off  OutDataTypeStr=boolean
  Accumulator Controller : MATLAB Function  TreatAsAtomicUnit=on
  Accumulator with Switches : Subsystem
  Compare To Constant1 : simulink/Logic and Bit Operations/Compare To Constant  relop===  const=nTheta-1  OutDataTypeStr=boolean
  Compare To Constant2 : simulink/Logic and Bit Operations/Compare To Constant  relop===  const=nRho-1  OutDataTypeStr=boolean
  Constant : Constant  Value=0  OutDataTypeStr=fixdt(0, ceil(log2(2*maxRho)), 0)  SampleTime=-1
  Constant1 : Constant  Value=nTheta-1  OutDataTypeStr=uint16  SampleTime=-1
  Constant2 : Constant  Value=nRho-1  OutDataTypeStr=uint16  SampleTime=-1
  Delay{1..4} (4 alike) : Delay  DelayLength=1
  Multiport Switch2 : MultiPortSwitch  DataPortOrder=Zero-based contiguous  Inputs=2  zeroidx=on
  Terminator : Terminator
  m_axis_tvalid : Outport
  m_axis_tdata : Outport  Port=2
  m_axis_tlast : Outport  Port=3
  wires:
  s_axis_tlast/1 -> Accumulator Controller/2(eof)
  Accumulator Controller/6(debug_state) -> Terminator/1
  Delay4/1 -> Multiport Switch2/1
  Delay2/1 -> m_axis_tvalid/1
  Accumulator Controller/5(valid) -> Delay2/1
  Constant/1 -> Multiport Switch2/3
  Accumulator with Switches/1(hps) -> Multiport Switch2/2
  Multiport Switch2/1 -> m_axis_tdata/1
  s_axis_tvalid/1 -> AND1/1
  AND1/1 -> Accumulator with Switches/2(edge)
  s_axis_tdata/1 -> AND1/2
  hough_param/1 -> Accumulator with Switches/1(hough_address)
  s_axis_tuser/1 -> Accumulator Controller/1(sof)
  Constant2/1 -> Accumulator Controller/4(nrho)
  Compare To Constant2/1 -> Delay3/1
  Accumulator Controller/4(index) -> Compare To Constant1/1, Accumulator with Switches/6(theta_index)
  Constant1/1 -> Accumulator Controller/3(ntheta)
  Accumulator Controller/2(read) -> Accumulator with Switches/4(read_address), Compare To Constant2/1
  Accumulator Controller/1(mode) -> Accumulator with Switches/3(mode), Delay4/1
  Accumulator Controller/3(clear) -> Accumulator with Switches/5(clear)
  Compare To Constant1/1 -> Delay1/1
  Delay3/1 -> AND/2
  Delay1/1 -> AND/1
  AND/1 -> m_axis_tlast/1

== system arlht_1920_1080/DUT/LHT/Parallel LHT Kernel ==
  s_tdata : Inport
  s_tvalid : Inport  Port=2
  s_tlast : Inport  Port=3
  AND : Logic  Inputs=3  IconShape=distinctive  AllPortsSameDT=off  OutDataTypeStr=boolean
  Bit Slice : hdlsllib/Logic and Bit Operations/Bit Slice  lidx=0  ridx=0
      settings: SourceProductBaseCode=SL
  Compare To Constant : simulink/Logic and Bit Operations/Compare To Constant  relop===  const=-width/2  OutDataTypeStr=boolean
  Compare To Constant1 : simulink/Logic and Bit Operations/Compare To Constant  relop===  const=-height/2  OutDataTypeStr=boolean
  Coordinate Counters : Subsystem
  Efficient Hough Kernel : Subsystem  mask{height=height, width=width}
      mask prompts: height "Image Height:"; width "Image Width:"
      mask init:
      | theta = [0:1:179];
      | 
      | maxRho = ceil(sqrt((height/2)^2+(width/2)^2));
      | [~, nTheta] = size(theta);
      | nRho = maxRho*2;
      mask DialogControl DescGroupVar Prompt: Efficient Hough Kernel
      mask DialogControl DescTextVar Prompt: The efficient Hough kernel uses look ahead and symmetric techniques to optimise DSP consumption.
  m_axis_tvalid : Outport  VectorParamsAs1DForOutWhenUnconnected=off
  m_axis_tdata : Outport  Port=2  VectorParamsAs1DForOutWhenUnconnected=off
  m_axis_tuser : Outport  Port=3  VectorParamsAs1DForOutWhenUnconnected=off
  m_axis_tlast : Outport  Port=4  VectorParamsAs1DForOutWhenUnconnected=off
  hough_param : Outport  Port=5  VectorParamsAs1DForOutWhenUnconnected=off
  wires:
  s_tlast/1 -> m_axis_tlast/1
  Compare To Constant/1 -> AND/2
  AND/1 -> m_axis_tuser/1
  Coordinate Counters/1(x) -> Compare To Constant/1, Efficient Hough Kernel/1(x)
  s_tvalid/1 -> m_axis_tvalid/1, AND/1, Coordinate Counters/1(valid)
  Coordinate Counters/2(y) -> Compare To Constant1/1, Efficient Hough Kernel/2(y)
  Compare To Constant1/1 -> AND/3
  Efficient Hough Kernel/1(rho) -> hough_param/1
  s_tdata/1 -> Bit Slice/1
  Bit Slice/1 -> m_axis_tdata/1

== system arlht_1920_1080/Memory Arrays/Accumulator Circuit/Accumulator Memory ==
  Edge : Inport
  Valid In : Inport  Port=2
  Mode : Inport  Port=3
  Address : Inport  Port=4
  Clear : Inport  Port=5
  AND1 : Logic  IconShape=distinctive  AllPortsSameDT=off  OutDataTypeStr=boolean
  Accumulator Memory : Subsystem
  Multiport Switch2 : MultiPortSwitch  DataPortOrder=Zero-based contiguous  Inputs=2  zeroidx=on
  HPS : Outport
  wires:
  Mode/1 -> Multiport Switch2/1, Accumulator Memory/1(Mode)
  Multiport Switch2/1 -> Accumulator Memory/3(Enable)
  Address/1 -> Accumulator Memory/2(Address)
  Valid In/1 -> AND1/2
  Accumulator Memory/1(HPS) -> HPS/1
  AND1/1 -> Multiport Switch2/3
  Edge/1 -> AND1/1
  Clear/1 -> Multiport Switch2/2

== system arlht_1920_1080/Memory Arrays/RBM Circuit/RBM Controller ==
  Magnitude : Inport
  Adjusted Orientation : Inport  Port=2
  Edge : Inport  Port=3
  Valid In : Inport  Port=4
  EoF In : Inport  Port=5
  Out1 : Outport
  y : Outport  Port=2
  Out2 : Outport  Port=3
  Valid Out : Outport  Port=4
  EoF Out : Outport  Port=5

== system arlht_1920_1080/Memory Arrays/RBM Circuit/RBM Memory ==
  mode : Inport
  address : Inport  Port=2
  enable : Inport  Port=3
  hps : Outport

== system arlht_1920_1080/DUT/LHT/Parallel LHT Accumulator/Accumulator with Switches ==
  hough_address : Inport
  edge : Inport  Port=2
  mode : Inport  Port=3
  read_address : Inport  Port=4
  clear : Inport  Port=5
  theta_index : Inport  Port=6
  Accumulator : Subsystem
  Data Type Conversion : DataTypeConversion  OutDataTypeStr=fixdt(0,ceil(log2(maxRho*2)),0)
  Delay : Delay  DelayLength=1
  Multiport Switch1 : MultiPortSwitch  DataPortOrder=Zero-based contiguous  Inputs=2  zeroidx=on
  Selector : Selector  NumberOfDimensions=2  IndexMode=Zero-based  InputPortWidth=3  IndexOptions=Index vector (dialog),Index vector (port)  Indices=0,0  OutputSizes=1,1
  Switch : Switch  Criteria=u2 > Threshold
  hps : Outport
  wires:
  Delay/1 -> Selector/2
  Data Type Conversion/1 -> Switch/3
  clear/1 -> Multiport Switch1/2
  edge/1 -> Multiport Switch1/3
  Selector/1 -> hps/1
  theta_index/1 -> Delay/1
  hough_address/1 -> Switch/1
  Multiport Switch1/1 -> Accumulator/3(edge)
  Switch/1 -> Accumulator/2(address)
  read_address/1 -> Data Type Conversion/1
  mode/1 -> Accumulator/1(mode), Multiport Switch1/1, Switch/2
  Accumulator/1(hps) -> Selector/1

== system arlht_1920_1080/DUT/LHT/Parallel LHT Kernel/Coordinate Counters ==
  valid : Inport
  AND : Logic  IconShape=distinctive  AllPortsSameDT=off  OutDataTypeStr=boolean
  Compare To Constant : simulink/Logic and Bit Operations/Compare To Constant  relop===  const=width/2-1  OutDataTypeStr=boolean
  X Counter : hdlsllib/Sources/HDL Counter  CountType=Count limited  CountInit=-width/2  CountStep=1  CountMax=width/2-1  CountFromType=Initial value  CountFrom=-width/2  CountResetPort=off  CountLoadPort=off  CountEnbPort=on  CountDirPort=off  CountDataType=Signed  CountWordLen=ceil(log2(width/2)) + 1  CountFracLen=0  CountSampTime=1
  Y Counter : hdlsllib/Sources/HDL Counter  CountType=Count limited  CountInit=-height/2  CountStep=1  CountMax=height/2-1  CountFromType=Initial value  CountFrom=-height/2  CountResetPort=off  CountLoadPort=off  CountEnbPort=on  CountDirPort=off  CountDataType=Signed  CountWordLen=ceil(log2(height/2)) + 1  CountFracLen=0  CountSampTime=1
  x : Outport  VectorParamsAs1DForOutWhenUnconnected=off
  y : Outport  Port=2  VectorParamsAs1DForOutWhenUnconnected=off
  wires:
  valid/1 -> AND/2, X Counter/1
  X Counter/1 -> x/1, Compare To Constant/1
  Y Counter/1 -> y/1
  AND/1 -> Y Counter/1
  Compare To Constant/1 -> AND/1

== system arlht_1920_1080/DUT/LHT/Parallel LHT Kernel/Efficient Hough Kernel ==
  x : Inport
  y : Inport  Port=2
  Add : Sum  OutDataTypeStr=fixdt(0, ceil(log2(2*maxRho+1)), 0)  RndMeth=Round
  Constant : Constant  Value=maxRho  OutDataTypeStr=fixdt(0, ceil(log2(maxRho + 1)), 0)  SampleTime=-1
  Look Ahead Hough : Subsystem
  Symmetric Kernel : Subsystem
  rho : Outport  VectorParamsAs1DForOutWhenUnconnected=off
  wires:
  Look Ahead Hough/1(ysin) -> Symmetric Kernel/2(ysin)
  y/1 -> Look Ahead Hough/2(y)
  Symmetric Kernel/1(rho) -> Add/2
  Add/1 -> rho/1
  Constant/1 -> Add/1
  x/1 -> Symmetric Kernel/1(x), Look Ahead Hough/1(x)

== system arlht_1920_1080/Memory Arrays/Accumulator Circuit/Accumulator Memory/Accumulator Memory ==
  Mode : Inport
  Address : Inport  Port=2
  Enable : Inport  Port=3
  AND : Logic  IconShape=distinctive  AllPortsSameDT=off  OutDataTypeStr=boolean
  Add : Sum  OutDataTypeStr=fixdt(0,bitsRho,0)
  Constant : Constant  OutDataTypeStr=fixdt(0,1,0)  SampleTime=-1
  Constant1 : Constant  Value=0  OutDataTypeStr=fixdt(0,bitsRho,0)  SampleTime=-1
  Delay{,1..3} (4 alike) : Delay  DelayLength=1
  Multiport Switch : MultiPortSwitch  DataPortOrder=Zero-based contiguous  Inputs=2  zeroidx=on
  Multiport Switch1 : MultiPortSwitch  DataPortOrder=Zero-based contiguous  Inputs=2  zeroidx=on
  Relational Operator : RelationalOperator  Operator===  OutDataTypeStr=boolean  RndMeth=Simplest
  Simple Dual Port RAM : hdlsllib/HDL RAMs/Simple Dual Port RAM  ram_size=ceil(log2(maxRho*2*180/Ktheta))
      settings: SourceProductBaseCode=SL
  HPS : Outport
  wires:
  Mode/1 -> Multiport Switch1/1
  Multiport Switch1/1 -> Simple Dual Port RAM/1
  Address/1 -> Relational Operator/2, Simple Dual Port RAM/4, Delay2/1
  Simple Dual Port RAM/1 -> HPS/1, Multiport Switch/2
  AND/1 -> Delay1/1
  Delay/1 -> Multiport Switch/3
  Multiport Switch/1 -> Add/2
  Delay2/1 -> Relational Operator/1, Simple Dual Port RAM/2
  Constant/1 -> Add/1
  Constant1/1 -> Multiport Switch1/2
  Add/1 -> Multiport Switch1/3, Delay/1
  Delay3/1 -> AND/1, Simple Dual Port RAM/3
  Relational Operator/1 -> AND/2
  Enable/1 -> Delay3/1
  Delay1/1 -> Multiport Switch/1

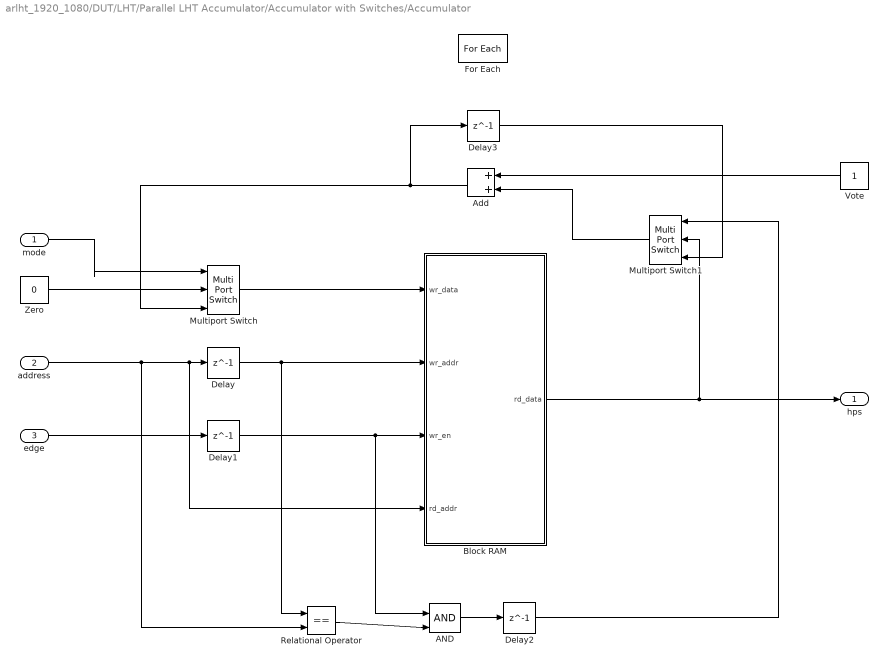
== system arlht_1920_1080/DUT/LHT/Parallel LHT Accumulator/Accumulator with Switches/Accumulator ==
  mode : Inport
  address : Inport  Port=2  Partition=on  PartitionDimension=2  PartitionWidth=1  PartitionOffset=0
  edge : Inport  Port=3
  AND : Logic  IconShape=distinctive  AllPortsSameDT=off  OutDataTypeStr=boolean
  Add : Sum  OutDataTypeStr=fixdt(0, ceil(log2(maxRho*2)), 0)
  Block RAM : Subsystem  Variant=on  VariantControlMode=Label  VariantControl=Variant1  LabelModeActiveChoice=other_bits
  Delay{,1..3} (4 alike) : Delay  DelayLength=1
  For Each : ForEach  DisableCoverage=on
  Multiport Switch : MultiPortSwitch  DataPortOrder=Zero-based contiguous  Inputs=2  zeroidx=on
  Multiport Switch1 : MultiPortSwitch  DataPortOrder=Zero-based contiguous  Inputs=2  zeroidx=on
  Relational Operator : RelationalOperator  Operator===  OutDataTypeStr=boolean  RndMeth=Simplest
  Vote : Constant  OutDataTypeStr=fixdt(0,1,0)  SampleTime=-1
  Zero : Constant  Value=0  OutDataTypeStr=fixdt(0,1,0)  SampleTime=-1
  hps : Outport  ConcatenationDimension=2
  wires:
  Block RAM/1(rd_data) -> hps/1, Multiport Switch1/2
  Multiport Switch/1 -> Block RAM/1(wr_data)
  mode/1 -> Multiport Switch/1
  edge/1 -> Delay1/1
  Zero/1 -> Multiport Switch/2
  Delay3/1 -> Multiport Switch1/3
  Vote/1 -> Add/1
  Multiport Switch1/1 -> Add/2
  Add/1 -> Delay3/1, Multiport Switch/3
  Delay1/1 -> Block RAM/3(wr_en), AND/1
  AND/1 -> Delay2/1
  address/1 -> Relational Operator/2, Delay/1, Block RAM/4(rd_addr)
  Delay2/1 -> Multiport Switch1/1
  Delay/1 -> Block RAM/2(wr_addr), Relational Operator/1
  Relational Operator/1 -> AND/2

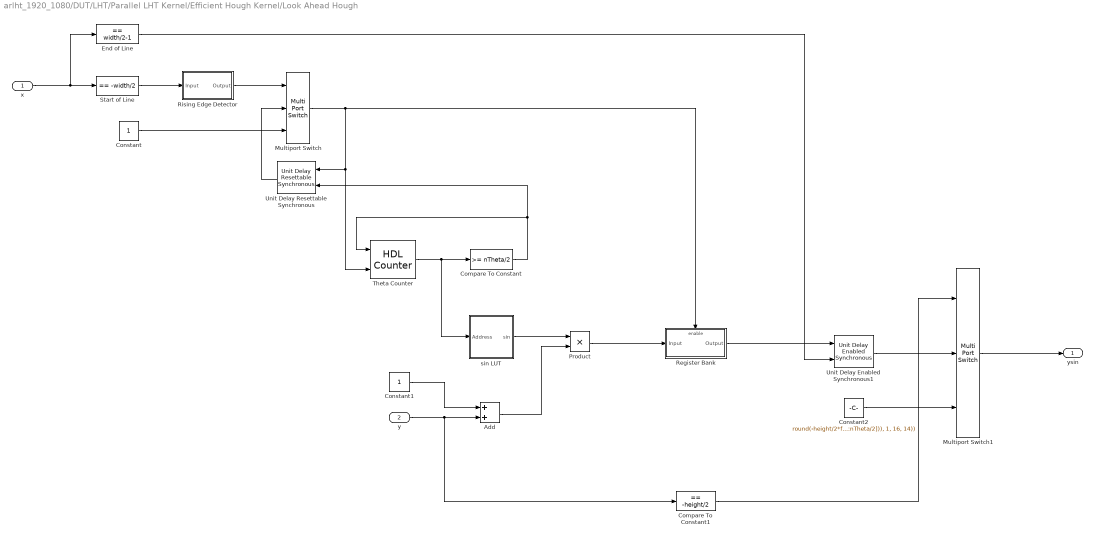
== system arlht_1920_1080/DUT/LHT/Parallel LHT Kernel/Efficient Hough Kernel/Look Ahead Hough ==
  x : Inport
  y : Inport  Port=2
  Add : Sum  OutDataTypeStr=fixdt(1,ceil(log2(height)),0)
  Compare To Constant : simulink/Logic and Bit Operations/Compare To Constant  relop=>=  const=nTheta/2  OutDataTypeStr=boolean
  Compare To Constant1 : simulink/Logic and Bit Operations/Compare To Constant  relop===  const=-height/2  OutDataTypeStr=boolean
  Constant : Constant  OutDataTypeStr=boolean  SampleTime=-1
  Constant1 : Constant  OutDataTypeStr=fixdt(1, ceil(log2(height)), 0);  SampleTime=-1
  Constant2 : Constant  Value=round(-height/2*fi(sin(deg2rad([0:1:nTheta/2])), 1, 16, 14))  OutDataTypeStr=fixdt(1,ceil(log2(height)),0)  SampleTime=-1
  End of Line : simulink/Logic and Bit Operations/Compare To Constant  relop===  const=width/2-1  OutDataTypeStr=boolean
  Multiport Switch : MultiPortSwitch  DataPortOrder=Zero-based contiguous  Inputs=2  zeroidx=on
  Multiport Switch1 : MultiPortSwitch  DataPortOrder=Zero-based contiguous  Inputs=2  zeroidx=on
  Product : Product  OutDataTypeStr=fixdt(1, ceil(log2(height)), 0);  RndMeth=Round
  Register Bank : Subsystem
  Rising Edge Detector : Subsystem
  Start of Line : simulink/Logic and Bit Operations/Compare To Constant  relop===  const=-width/2  OutDataTypeStr=boolean
  Theta Counter : hdlsllib/Sources/HDL Counter  CountType=Count limited  CountInit=0  CountStep=1  CountMax=nTheta/2  CountFromType=Initial value  CountFrom=0  CountResetPort=on  CountLoadPort=off  CountEnbPort=on  CountDirPort=off  CountDataType=Unsigned  CountWordLen=ceil(log2(nTheta))  CountFracLen=0  CountSampTime=1
  Unit Delay Enabled Synchronous1 : hdlsllib/Discrete/Unit Delay Enabled Synchronous  InitialCondition=0.0  SampleTime=-1
      settings: SourceProductBaseCode=SL
  Unit Delay Resettable Synchronous : hdlsllib/Discrete/Unit Delay Resettable Synchronous  InitialCondition=0.0  SampleTime=-1
      settings: SourceProductBaseCode=SL
  sin LUT : Subsystem
  ysin : Outport  VectorParamsAs1DForOutWhenUnconnected=off
  wires:
  x/1 -> End of Line/1, Start of Line/1
  Start of Line/1 -> Rising Edge Detector/1(Input)
  Multiport Switch/1 -> Register Bank/Enable, Unit Delay Resettable Synchronous/1, Theta Counter/2
  Unit Delay Resettable Synchronous/1 -> Multiport Switch/2
  Constant/1 -> Multiport Switch/3
  Theta Counter/1 -> sin LUT/1(Address), Compare To Constant/1
  Constant1/1 -> Add/1
  Rising Edge Detector/1(Output) -> Multiport Switch/1
  Add/1 -> Product/2
  Multiport Switch1/1 -> ysin/1
  Constant2/1 -> Multiport Switch1/3
  Compare To Constant1/1 -> Multiport Switch1/1
  Product/1 -> Register Bank/1(Input)
  y/1 -> Add/2, Compare To Constant1/1
  Compare To Constant/1 -> Unit Delay Resettable Synchronous/2, Theta Counter/1
  Unit Delay Enabled Synchronous1/1 -> Multiport Switch1/2
  End of Line/1 -> Unit Delay Enabled Synchronous1/2
  Register Bank/1(Output) -> Unit Delay Enabled Synchronous1/1
  sin LUT/1(sin) -> Product/1
